simulink model "Subsystem"  (R2016a)
settings: Solver=FixedStepDiscrete  StartTime=0.0  StopTime=10.0  RelTol=1e-3
values from neighbouring files (symbols this model uses):
  a1 = 1    [Prob_7_mat.mat]
  a2 = 2    [Prob_7_mat.mat]
  a3 = 3    [Prob_7_mat.mat]
  a4 = 1    [Prob_7_mat.mat]
  a5 = 1    [Prob_7_mat.mat]
  a6 = 1    [Prob_7_mat.mat]
settings Model: Creator=Admin  LastModifiedBy=Admin
settings DataIOCC: SaveOutput=off  SaveTime=off

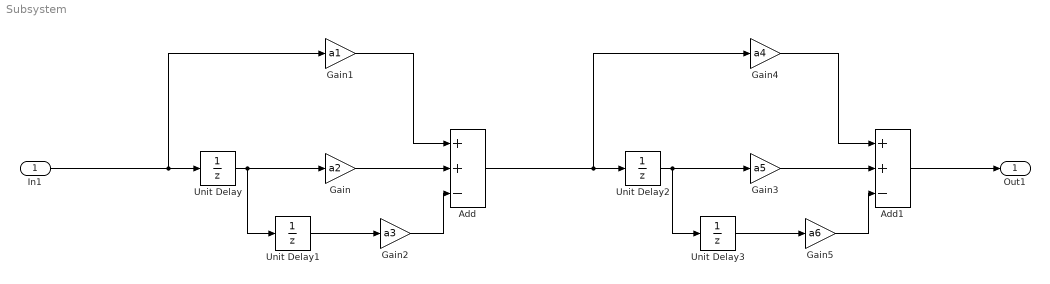
== system Subsystem ==
  In1 : Inport  OutDataTypeStr=double  PortDimensions=1  SampleTime=0
  Add : Sum  Inputs=++-
  Add1 : Sum  Inputs=++-
  Gain : Gain  Gain=a2
  Gain1 : Gain  Gain=a1
  Gain2 : Gain  Gain=a3
  Gain3 : Gain  Gain=a5
  Gain4 : Gain  Gain=a4
  Gain5 : Gain  Gain=a6
  Unit Delay{,1..3} (4 alike) : UnitDelay  SampleTime=-1
  Out1 : Outport  OutDataTypeStr=double  PortDimensions=1  SampleTime=0
  wires:
  Unit Delay/1 -> Gain/1, Unit Delay1/1
  Gain1/1 -> Add/1
  In1/1 -> Gain1/1, Unit Delay/1
  Add1/1 -> Out1/1
  Gain3/1 -> Add1/2
  Gain2/1 -> Add/3
  Unit Delay1/1 -> Gain2/1
  Add/1 -> Gain4/1, Unit Delay2/1
  Unit Delay3/1 -> Gain5/1
  Unit Delay2/1 -> Gain3/1, Unit Delay3/1
  Gain/1 -> Add/2
  Gain5/1 -> Add1/3
  Gain4/1 -> Add1/1
